simulink model "Single_Phase_Bridge_Rectifier_RL_Load"  (R2018a)
settings: Solver=VariableStepAuto  StartTime=0.0  StopTime=0.1  RelTol=1e-3
libraries: powerlib x13, powerlib_meascontrol x5
settings Model: Creator=ozie  LastModifiedBy=ozie

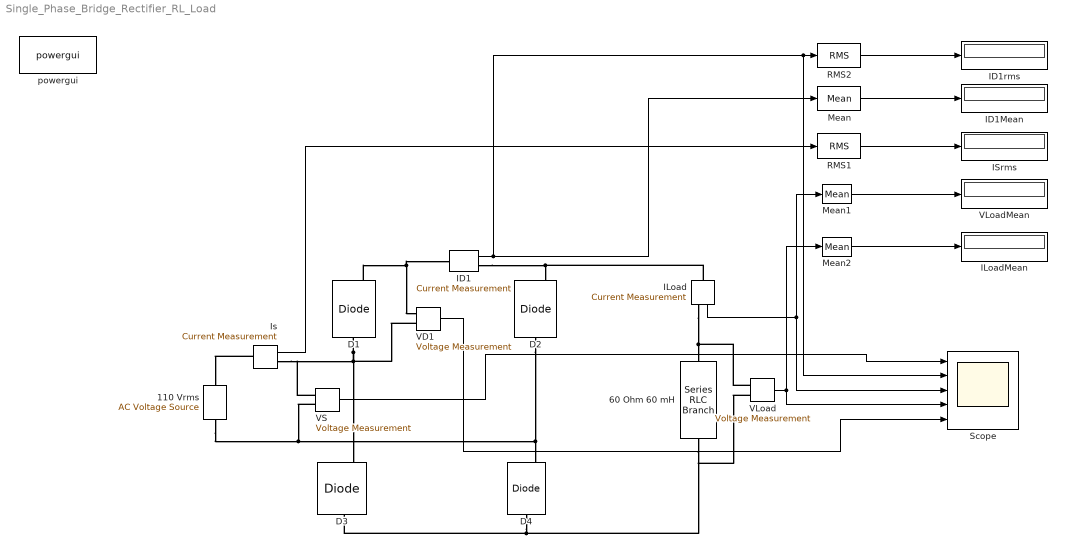
== system Single_Phase_Bridge_Rectifier_RL_Load ==
  110 Vrms : powerlib/Electrical Sources/AC Voltage Source  Amplitude=110*sqrt(2)  Phase=0  Frequency=50  SampleTime=0  Measurements=None  BusType=swing  Pref=10e3  Qref=0  Qmin=-inf  Qmax=+inf
  60 Ohm 60 mH : powerlib/Elements/Series RLC Branch  LConnTagsString=__new0  RConnTagsString=__new0  BranchType=RL  Resistance=60  Inductance=60e-3  SetiL0=off  InitialCurrent=0  Capacitance=1e-6  Setx0=off  InitialVoltage=0  Measurements=None
  D{1..4} (4 alike) : powerlib/Power Electronics/Diode  Ron=0.001  Lon=0  Vf=0.8  IC=0  UseSnubber=0  Rs=500  Cs=250e-9  Measurements=on
  ID1 : powerlib/Measurements/Current Measurement  PhasorSimulation=off  OutputType=Complex  PSBequivalent=0
  ID1Mean : Display
  ID1rms : Display
  ILoad : powerlib/Measurements/Current Measurement  PhasorSimulation=off  OutputType=Complex  PSBequivalent=0
  "ILoadMean " : Display
  ISrms : Display
  Is : powerlib/Measurements/Current Measurement  PhasorSimulation=off  OutputType=Complex  PSBequivalent=0
  Mean : powerlib_meascontrol/Measurements/Mean  Freq=60  Vinit=0  Ts=0
  Mean1 : powerlib_meascontrol/Measurements/Mean  Freq=50  Vinit=0  Ts=0
  Mean2 : powerlib_meascontrol/Measurements/Mean  Freq=50  Vinit=0  Ts=0
  RMS1 : powerlib_meascontrol/Measurements/RMS  TrueRMS=on  Freq=60  RMSInit=120  Ts=0
  RMS2 : powerlib_meascontrol/Measurements/RMS  TrueRMS=on  Freq=60  RMSInit=120  Ts=0
  Scope : Scope  NumInputPorts=5
  "VD1 " : powerlib/Measurements/Voltage Measurement  PhasorSimulation=off  OutputType=Complex  PSBequivalent=0
  VLoad : powerlib/Measurements/Voltage Measurement  PhasorSimulation=off  OutputType=Complex  PSBequivalent=0
  VLoadMean : Display
  VS : powerlib/Measurements/Voltage Measurement  PhasorSimulation=off  OutputType=Complex  PSBequivalent=0
  powergui : powerlib/powergui  Priority=1  SimulationMode=Continuous  SampleTime=50e-6  frequency=60  Iterations=50  frequencyindice=50  Pbase=100e6  ErrMax=1e-4  UnitsV=kV  UnitsW=MW  buscounter=0  FunctionMessages=off  echomessages=off  EnableUseOfTLC=off  CurrentSourceSwitches=off  DisableSnubberDevices=off  DisableRonSwitches=off  DisableVfSwitches=off  DisplayEquations=off  SolverType=Tustin/Backward Euler (TBE)  Interpol=off  ExternalGateDelay=off  methode=off  Ts=100  x0status=blocks  SPID=on  SwTol=0  HookPort=off  RestoreLinks=warning  ResistiveCurrentMeasurement=off  Frange=[0:2:500]  Ylog=off  Xlog=on  ShowGrid=off  save=off  variable=ZData  structure=0  ZoomFFT=off  StartTime=0.0  cycles=1  DisplayStyle=1  fundamental=60  FreqAxis=off  MaxFrequency=1000  frequencyindicesteady=1  RmsSteady=1  display=off
  wires:
  Mean/1 -> ID1Mean/1
  RMS1/1 -> ISrms/1
  Is/1 -> RMS1/1
  ID1/1 -> Scope/2, RMS2/1, Mean/1
  Mean1/1 -> VLoadMean/1
  ILoad/1 -> Scope/3, Mean1/1
  Mean2/1 -> "ILoadMean "/1
  VLoad/1 -> Scope/4, Mean2/1
  RMS2/1 -> ID1rms/1
  VS/1 -> Scope/1
  "VD1 "/1 -> Scope/5
  connections:
  D1/LConn1 -- Is/RConn1 -- VS/LConn1 -- "VD1 "/LConn1 -- D3/RConn1
  110 Vrms/LConn1 -- VS/LConn2 -- D2/LConn1 -- D4/RConn1
  D4/LConn1 -- VLoad/LConn2 -- 60 Ohm 60 mH/RConn1 -- D3/LConn1
  D1/RConn1 -- "VD1 "/LConn2 -- ID1/LConn1
  ILoad/RConn1 -- VLoad/LConn1 -- 60 Ohm 60 mH/LConn1
  Is/LConn1 -- 110 Vrms/RConn1
  ILoad/LConn1 -- ID1/RConn1 -- D2/RConn1
